simulink model "Room_model_without_subsystem_2015a"  (R2015a)
settings: Solver=ode45  StartTime=0.0  StopTime=Inf  RelTol=1e-3
InitFcn:
  | server = Sim_server(10000);
StopFcn:
  | server.stop
values from neighbouring files (symbols this model uses):
  Cth = 1300    [Room_Model_Variables.m]
  Rth = 1/0.8    (= 1.25)    [Room_Model_Variables.m]
  x1 = 1    [Room_Model_Variables.m]
  x2 = 1    [Room_Model_Variables.m]
  x3 = 1    [Room_Model_Variables.m]
  y1 = 1    [Room_Model_Variables.m]
  y2 = 1    [Room_Model_Variables.m]
  y3 = 1    [Room_Model_Variables.m]
libraries: simulink x1
settings Model: CovModelRefEnable=off  Creator=e0154145  LastModifiedBy=accma
settings DataIOCC: LimitDataPoints=off  SaveFormat=Dataset
settings HardwareCC: ProdBitPerPointer=64  ProdLargestAtomicFloat=Float  ProdIntDivRoundTo=Zero  ProdEndianess=LittleEndian  ProdHWDeviceType=Specified
settings ModelReferenceCC: PropagateSignalLabelsOutOfModel=on

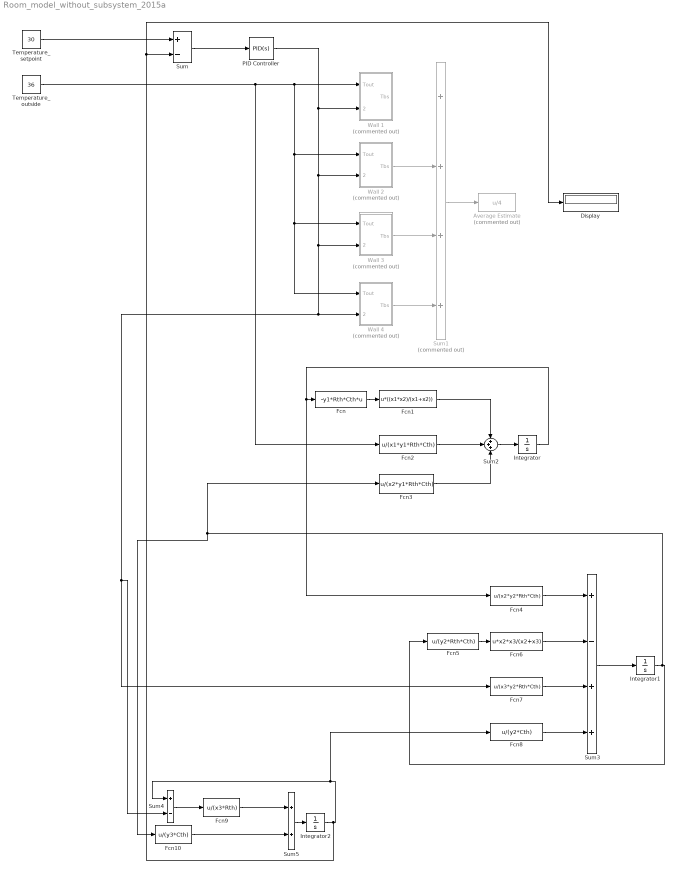
== system Room_model_without_subsystem_2015a ==
  Average Estimate : Fcn  Commented=on  Expr=u/4
  Display : Display
  Fcn : Fcn  Expr=-y1*Rth*Cth*u
  Fcn1 : Fcn  Expr=u*((x1*x2)/(x1+x2))
  Fcn10 : Fcn  Expr=u/(y3*Cth)
  Fcn2 : Fcn  Expr=u/(x1*y1*Rth*Cth)
  Fcn3 : Fcn  Expr=u/(x2*y1*Rth*Cth)
  Fcn4 : Fcn  Expr=u/(x2*y2*Rth*Cth)
  Fcn5 : Fcn  Expr=u/(y2*Rth*Cth)
  Fcn6 : Fcn  Expr=u*x2*x3/(x2+x3)
  Fcn7 : Fcn  Expr=u/(x3*y2*Rth*Cth)
  Fcn8 : Fcn  Expr=u/(y2*Cth)
  Fcn9 : Fcn  Expr=u/(x3*Rth)
  Integrator : Integrator
  Integrator1 : Integrator
  Integrator2 : Integrator
  PID Controller : simulink/Continuous/PID Controller  Controller=PID  TimeDomain=Continuous-time  SampleTime=-1  IntegratorMethod=Forward Euler  FilterMethod=Forward Euler  Form=Parallel  UseFilter=on  ControllerParametersSource=internal  P=-48.5287946828106  I=-345.034799736216  D=-0.161133654003053  N=216.924955724861  InitialConditionSource=internal  InitialConditionForIntegrator=0  InitialConditionForFilter=0  ExternalReset=none  LimitOutput=off  UpperSaturationLimit=inf  LowerSaturationLimit=-inf  LinearizeAsGain=on  AntiWindupMode=none  Kb=1  TrackingMode=off  Kt=1  PParamMin=[]  PParamMax=[]  IParamMin=[]  IParamMax=[]  DParamMin=[]  DParamMax=[]  NParamMin=[]  NParamMax=[]  KbParamMin=[]  KbParamMax=[]  KtParamMin=[]  KtParamMax=[]  POutMin=[]  POutMax=[]  IOutMin=[]  IOutMax=[]  DOutMin=[]  DOutMax=[]  NOutMin=[]  NOutMax=[]  KbOutMin=[]  KbOutMax=[]  KtOutMin=[]  KtOutMax=[]  IntegratorOutMin=[]  IntegratorOutMax=[]  FilterOutMin=[]  FilterOutMax=[]  SumOutMin=[]  SumOutMax=[]  SumI1OutMin=[]  SumI1OutMax=[]  SumI2OutMin=[]  SumI2OutMax=[]  SumI3OutMin=[]  SumI3OutMax=[]  SumDOutMin=[]  SumDOutMax=[]  SaturationOutMin=[]  SaturationOutMax=[]  IntegratorContinuousStateAttributes=''  IntegratorStateMustResolveToSignalObject=off  IntegratorRTWStateStorageClass=Auto  FilterContinuousStateAttributes=''  FilterStateMustResolveToSignalObject=off  FilterRTWStateStorageClass=Auto  DifferentiatorICPrevScaledInput=0  DifferentiatorOutMin=[]  DifferentiatorOutMax=[]
  Sum : Sum  Inputs=+-
  Sum1 : Sum  Commented=on  Inputs=++++
  Sum2 : Sum  Inputs=3
  Sum3 : Sum  Inputs=+-++  RndMeth=Round
  Sum4 : Sum  Inputs=+-
  Sum5 : Sum
  Temperature_outside : Constant  Value=36
  Temperature_setpoint : Constant  Value=30  OutMin=[16]  OutMax=[30]
  "Wall 1 " : Subsystem  Commented=on
  Wall 2 : Subsystem  Commented=on
  Wall 3 : Subsystem  Commented=on
  Wall 4 : Subsystem  Commented=on
  wires:
  Temperature_setpoint/1 -> Sum/1
  Sum/1 -> PID Controller/1
  Wall 4/1("Tbs ") -> Sum1/4
  Wall 3/1("Tbs ") -> Sum1/3
  Sum1/1 -> Average Estimate/1
  Wall 2/1("Tbs ") -> Sum1/2
  Fcn3/1 -> Sum2/3
  Sum2/1 -> Integrator/1
  Fcn2/1 -> Sum2/2
  Fcn1/1 -> Sum2/1
  Fcn/1 -> Fcn1/1
  Temperature_outside/1 -> Fcn2/1, Wall 4/1(Tout), Wall 3/1(Tout), Wall 2/1(Tout), "Wall 1 "/1(Tout)
  Fcn5/1 -> Fcn6/1
  Sum3/1 -> Integrator1/1
  Integrator/1 -> Fcn4/1, Fcn/1
  Fcn6/1 -> Sum3/2
  Fcn8/1 -> Sum3/4
  Fcn7/1 -> Sum3/3
  Fcn4/1 -> Sum3/1
  Sum5/1 -> Integrator2/1
  Fcn9/1 -> Sum5/1
  Fcn10/1 -> Sum5/2
  Sum4/1 -> Fcn9/1
  Integrator1/1 -> Fcn5/1, Fcn3/1, Fcn10/1
  Integrator2/1 -> Display/1, Sum/2, Fcn8/1, Sum4/1
  PID Controller/1 -> Wall 4/2(Qhvac), Fcn7/1, Sum4/2, Wall 3/2(Qhvac), Wall 2/2(Qhvac), "Wall 1 "/2(Qhvac)

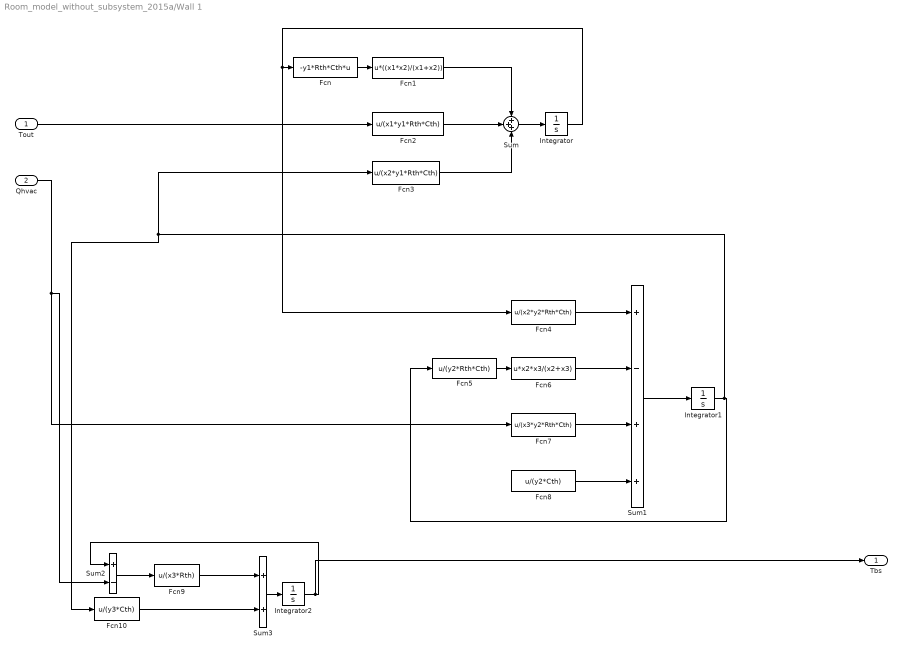
== system Room_model_without_subsystem_2015a/Wall 1  ==
  Tout : Inport
  Qhvac : Inport  Port=2
  Fcn : Fcn  Expr=-y1*Rth*Cth*u
  Fcn1 : Fcn  Expr=u*((x1*x2)/(x1+x2))
  Fcn10 : Fcn  Expr=u/(y3*Cth)
  Fcn2 : Fcn  Expr=u/(x1*y1*Rth*Cth)
  Fcn3 : Fcn  Expr=u/(x2*y1*Rth*Cth)
  Fcn4 : Fcn  Expr=u/(x2*y2*Rth*Cth)
  Fcn5 : Fcn  Expr=u/(y2*Rth*Cth)
  Fcn6 : Fcn  Expr=u*x2*x3/(x2+x3)
  Fcn7 : Fcn  Expr=u/(x3*y2*Rth*Cth)
  Fcn8 : Fcn  Expr=u/(y2*Cth)
  Fcn9 : Fcn  Expr=u/(x3*Rth)
  Integrator : Integrator
  Integrator1 : Integrator
  Integrator2 : Integrator
  Sum : Sum  Inputs=3
  Sum1 : Sum  Inputs=+-++  RndMeth=Round
  Sum2 : Sum  Inputs=+-
  Sum3 : Sum
  "Tbs " : Outport
  wires:
  Fcn3/1 -> Sum/3
  Sum/1 -> Integrator/1
  Fcn2/1 -> Sum/2
  Fcn1/1 -> Sum/1
  Fcn/1 -> Fcn1/1
  Tout/1 -> Fcn2/1
  Fcn5/1 -> Fcn6/1
  Sum1/1 -> Integrator1/1
  Integrator/1 -> Fcn4/1, Fcn/1
  Fcn6/1 -> Sum1/2
  Fcn8/1 -> Sum1/4
  Fcn7/1 -> Sum1/3
  Fcn4/1 -> Sum1/1
  Sum3/1 -> Integrator2/1
  Fcn9/1 -> Sum3/1
  Fcn10/1 -> Sum3/2
  Sum2/1 -> Fcn9/1
  Integrator1/1 -> Fcn5/1, Fcn3/1, Fcn10/1
  Integrator2/1 -> "Tbs "/1, Sum2/1
  Qhvac/1 -> Fcn7/1, Sum2/2

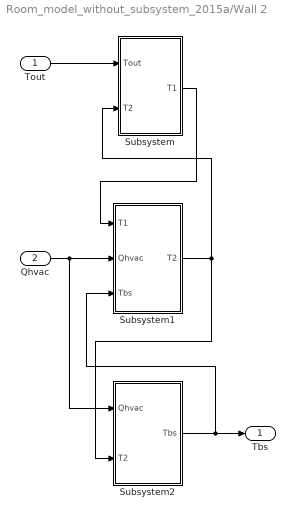
== system Room_model_without_subsystem_2015a/Wall 2 ==
  Tout : Inport
  Qhvac : Inport  Port=2
  Subsystem : Subsystem
  Subsystem1 : Subsystem
  Subsystem2 : Subsystem
  "Tbs " : Outport
  wires:
  Tout/1 -> Subsystem/1(Tout)
  Subsystem2/1("Tbs ") -> Subsystem1/3(Tbs), "Tbs "/1
  Subsystem/1(T1) -> Subsystem1/1("T1 ")
  Qhvac/1 -> Subsystem1/2(Qhvac), Subsystem2/1("Qhvac ")
  Subsystem1/1("T2 ") -> Subsystem2/2("T2 "), Subsystem/2(T2)

== system Room_model_without_subsystem_2015a/Wall 3 ==
  Tout : Inport
  Qhvac : Inport  Port=2
  Subsystem : Subsystem
  Subsystem1 : Subsystem
  Subsystem2 : Subsystem
  "Tbs " : Outport
  wires:
  Tout/1 -> Subsystem/1(Tout)
  Subsystem2/1("Tbs ") -> Subsystem1/3(Tbs), "Tbs "/1
  Subsystem/1(T1) -> Subsystem1/1("T1 ")
  Qhvac/1 -> Subsystem1/2(Qhvac), Subsystem2/1("Qhvac ")
  Subsystem1/1("T2 ") -> Subsystem2/2("T2 "), Subsystem/2(T2)

== system Room_model_without_subsystem_2015a/Wall 4 ==
  Tout : Inport
  Qhvac : Inport  Port=2
  Subsystem : Subsystem
  Subsystem1 : Subsystem
  Subsystem2 : Subsystem
  "Tbs " : Outport
  wires:
  Tout/1 -> Subsystem/1(Tout)
  Subsystem2/1("Tbs ") -> Subsystem1/3(Tbs), "Tbs "/1
  Subsystem/1(T1) -> Subsystem1/1("T1 ")
  Qhvac/1 -> Subsystem1/2(Qhvac), Subsystem2/1("Qhvac ")
  Subsystem1/1("T2 ") -> Subsystem2/2("T2 "), Subsystem/2(T2)

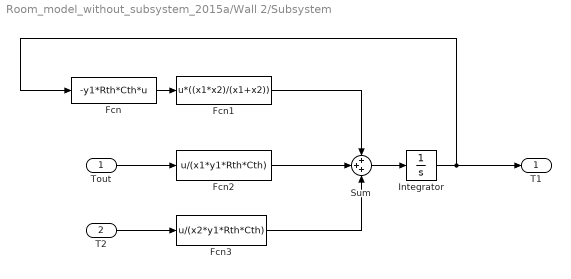
== system Room_model_without_subsystem_2015a/Wall 2/Subsystem ==
  Tout : Inport
  T2 : Inport  Port=2
  Fcn : Fcn  Expr=-y1*Rth*Cth*u
  Fcn1 : Fcn  Expr=u*((x1*x2)/(x1+x2))
  Fcn2 : Fcn  Expr=u/(x1*y1*Rth*Cth)
  Fcn3 : Fcn  Expr=u/(x2*y1*Rth*Cth)
  Integrator : Integrator
  Sum : Sum  Inputs=3
  T1 : Outport
  wires:
  T2/1 -> Fcn3/1
  Fcn3/1 -> Sum/3
  Sum/1 -> Integrator/1
  Fcn2/1 -> Sum/2
  Fcn1/1 -> Sum/1
  Integrator/1 -> T1/1, Fcn/1
  Fcn/1 -> Fcn1/1
  Tout/1 -> Fcn2/1

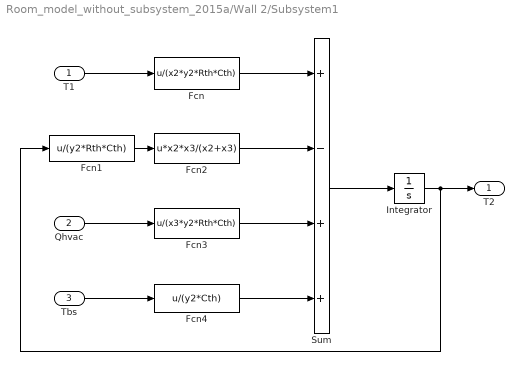
== system Room_model_without_subsystem_2015a/Wall 2/Subsystem1 ==
  "T1 " : Inport
  Qhvac : Inport  Port=2
  Tbs : Inport  Port=3
  Fcn : Fcn  Expr=u/(x2*y2*Rth*Cth)
  Fcn1 : Fcn  Expr=u/(y2*Rth*Cth)
  Fcn2 : Fcn  Expr=u*x2*x3/(x2+x3)
  Fcn3 : Fcn  Expr=u/(x3*y2*Rth*Cth)
  Fcn4 : Fcn  Expr=u/(y2*Cth)
  Integrator : Integrator
  Sum : Sum  Inputs=+-++  RndMeth=Round
  "T2 " : Outport
  wires:
  Fcn1/1 -> Fcn2/1
  Integrator/1 -> "T2 "/1, Fcn1/1
  Sum/1 -> Integrator/1
  "T1 "/1 -> Fcn/1
  Qhvac/1 -> Fcn3/1
  Fcn2/1 -> Sum/2
  Tbs/1 -> Fcn4/1
  Fcn4/1 -> Sum/4
  Fcn3/1 -> Sum/3
  Fcn/1 -> Sum/1

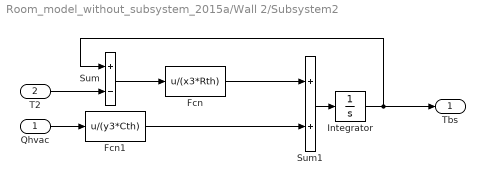
== system Room_model_without_subsystem_2015a/Wall 2/Subsystem2 ==
  "Qhvac " : Inport
  "T2 " : Inport  Port=2
  Fcn : Fcn  Expr=u/(x3*Rth)
  Fcn1 : Fcn  Expr=u/(y3*Cth)
  Integrator : Integrator
  Sum : Sum  Inputs=+-
  Sum1 : Sum
  "Tbs " : Outport
  wires:
  Sum1/1 -> Integrator/1
  Fcn/1 -> Sum1/1
  Fcn1/1 -> Sum1/2
  Sum/1 -> Fcn/1
  "Qhvac "/1 -> Fcn1/1
  Integrator/1 -> "Tbs "/1, Sum/1
  "T2 "/1 -> Sum/2

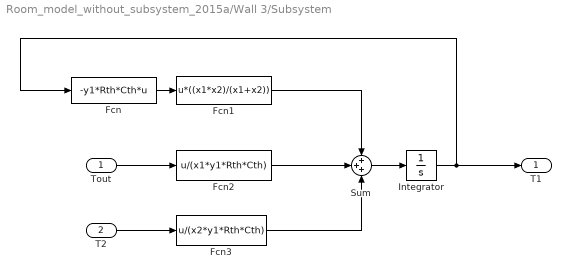
== system Room_model_without_subsystem_2015a/Wall 3/Subsystem ==
  Tout : Inport
  T2 : Inport  Port=2
  Fcn : Fcn  Expr=-y1*Rth*Cth*u
  Fcn1 : Fcn  Expr=u*((x1*x2)/(x1+x2))
  Fcn2 : Fcn  Expr=u/(x1*y1*Rth*Cth)
  Fcn3 : Fcn  Expr=u/(x2*y1*Rth*Cth)
  Integrator : Integrator
  Sum : Sum  Inputs=3
  T1 : Outport
  wires:
  T2/1 -> Fcn3/1
  Fcn3/1 -> Sum/3
  Sum/1 -> Integrator/1
  Fcn2/1 -> Sum/2
  Fcn1/1 -> Sum/1
  Integrator/1 -> T1/1, Fcn/1
  Fcn/1 -> Fcn1/1
  Tout/1 -> Fcn2/1

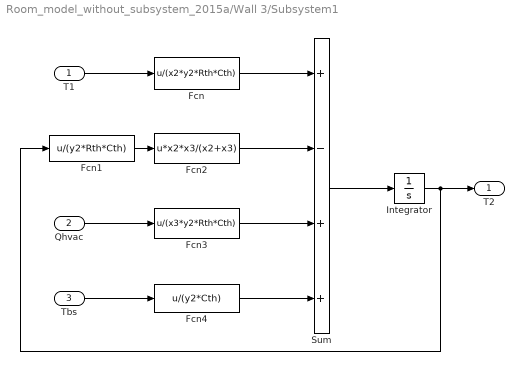
== system Room_model_without_subsystem_2015a/Wall 3/Subsystem1 ==
  "T1 " : Inport
  Qhvac : Inport  Port=2
  Tbs : Inport  Port=3
  Fcn : Fcn  Expr=u/(x2*y2*Rth*Cth)
  Fcn1 : Fcn  Expr=u/(y2*Rth*Cth)
  Fcn2 : Fcn  Expr=u*x2*x3/(x2+x3)
  Fcn3 : Fcn  Expr=u/(x3*y2*Rth*Cth)
  Fcn4 : Fcn  Expr=u/(y2*Cth)
  Integrator : Integrator
  Sum : Sum  Inputs=+-++  RndMeth=Round
  "T2 " : Outport
  wires:
  Fcn1/1 -> Fcn2/1
  Integrator/1 -> "T2 "/1, Fcn1/1
  Sum/1 -> Integrator/1
  "T1 "/1 -> Fcn/1
  Qhvac/1 -> Fcn3/1
  Fcn2/1 -> Sum/2
  Tbs/1 -> Fcn4/1
  Fcn4/1 -> Sum/4
  Fcn3/1 -> Sum/3
  Fcn/1 -> Sum/1

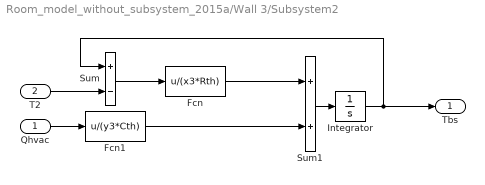
== system Room_model_without_subsystem_2015a/Wall 3/Subsystem2 ==
  "Qhvac " : Inport
  "T2 " : Inport  Port=2
  Fcn : Fcn  Expr=u/(x3*Rth)
  Fcn1 : Fcn  Expr=u/(y3*Cth)
  Integrator : Integrator
  Sum : Sum  Inputs=+-
  Sum1 : Sum
  "Tbs " : Outport
  wires:
  Sum1/1 -> Integrator/1
  Fcn/1 -> Sum1/1
  Fcn1/1 -> Sum1/2
  Sum/1 -> Fcn/1
  "Qhvac "/1 -> Fcn1/1
  Integrator/1 -> "Tbs "/1, Sum/1
  "T2 "/1 -> Sum/2

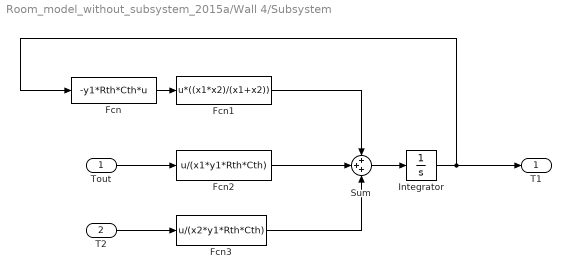
== system Room_model_without_subsystem_2015a/Wall 4/Subsystem ==
  Tout : Inport
  T2 : Inport  Port=2
  Fcn : Fcn  Expr=-y1*Rth*Cth*u
  Fcn1 : Fcn  Expr=u*((x1*x2)/(x1+x2))
  Fcn2 : Fcn  Expr=u/(x1*y1*Rth*Cth)
  Fcn3 : Fcn  Expr=u/(x2*y1*Rth*Cth)
  Integrator : Integrator
  Sum : Sum  Inputs=3
  T1 : Outport
  wires:
  T2/1 -> Fcn3/1
  Fcn3/1 -> Sum/3
  Sum/1 -> Integrator/1
  Fcn2/1 -> Sum/2
  Fcn1/1 -> Sum/1
  Integrator/1 -> T1/1, Fcn/1
  Fcn/1 -> Fcn1/1
  Tout/1 -> Fcn2/1

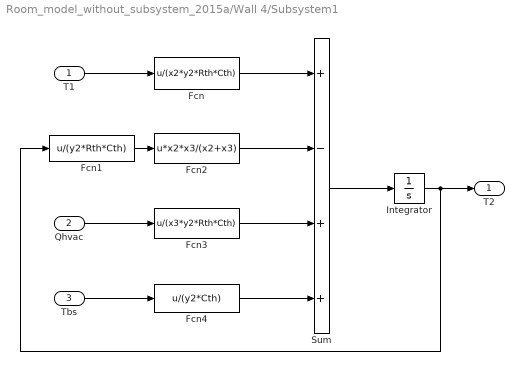
== system Room_model_without_subsystem_2015a/Wall 4/Subsystem1 ==
  "T1 " : Inport
  Qhvac : Inport  Port=2
  Tbs : Inport  Port=3
  Fcn : Fcn  Expr=u/(x2*y2*Rth*Cth)
  Fcn1 : Fcn  Expr=u/(y2*Rth*Cth)
  Fcn2 : Fcn  Expr=u*x2*x3/(x2+x3)
  Fcn3 : Fcn  Expr=u/(x3*y2*Rth*Cth)
  Fcn4 : Fcn  Expr=u/(y2*Cth)
  Integrator : Integrator
  Sum : Sum  Inputs=+-++  RndMeth=Round
  "T2 " : Outport
  wires:
  Fcn1/1 -> Fcn2/1
  Integrator/1 -> "T2 "/1, Fcn1/1
  Sum/1 -> Integrator/1
  "T1 "/1 -> Fcn/1
  Qhvac/1 -> Fcn3/1
  Fcn2/1 -> Sum/2
  Tbs/1 -> Fcn4/1
  Fcn4/1 -> Sum/4
  Fcn3/1 -> Sum/3
  Fcn/1 -> Sum/1

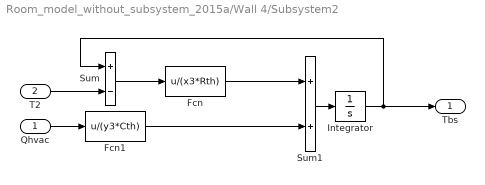
== system Room_model_without_subsystem_2015a/Wall 4/Subsystem2 ==
  "Qhvac " : Inport
  "T2 " : Inport  Port=2
  Fcn : Fcn  Expr=u/(x3*Rth)
  Fcn1 : Fcn  Expr=u/(y3*Cth)
  Integrator : Integrator
  Sum : Sum  Inputs=+-
  Sum1 : Sum
  "Tbs " : Outport
  wires:
  Sum1/1 -> Integrator/1
  Fcn/1 -> Sum1/1
  Fcn1/1 -> Sum1/2
  Sum/1 -> Fcn/1
  "Qhvac "/1 -> Fcn1/1
  Integrator/1 -> "Tbs "/1, Sum/1
  "T2 "/1 -> Sum/2
